simulink model "PMSM_FOC_CLOOP"  (R2022a)
settings: Solver=FixedStepAuto  StartTime=0.0  StopTime=0.5  FixedStep=Ts  RelTol=1e-3
undefined symbols (not defined in the file): Ki_C, Kp_C, pmsm, Ts
libraries: mcbcontrolslib x5, slpidlib x2, mcbplantlib x1, autolibpmsmexterior x1
settings Model: Creator=徐国强  LastModifiedBy=徐国强

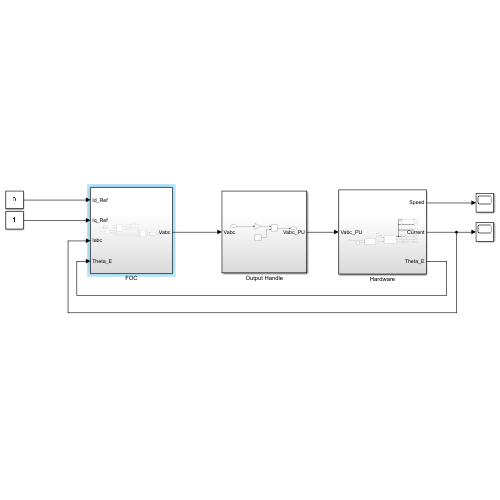
[thumbnail: Simulink's stored preview of the top-level diagram]
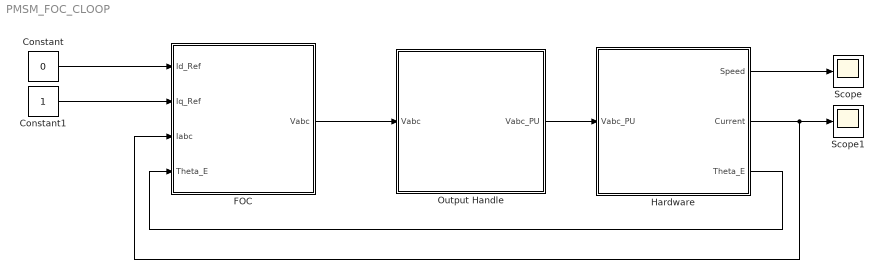
== system PMSM_FOC_CLOOP ==
  Constant : Constant  Value=0
  Constant1 : Constant
  FOC : Subsystem
  Hardware : Subsystem
  Output Handle : Subsystem
  Scope : Scope
  Scope1 : Scope
  wires:
  FOC/1(Vabc) -> Output Handle/1(Vabc)
  Output Handle/1(Vabc_PU) -> Hardware/1(Vabc_PU)
  Hardware/1(Speed) -> Scope/1
  Hardware/2(Current) -> FOC/3(Iabc), Scope1/1
  Hardware/3(Theta_E) -> FOC/4(Theta_E)
  Constant/1 -> FOC/1(Id_Ref)
  Constant1/1 -> FOC/2(Iq_Ref)

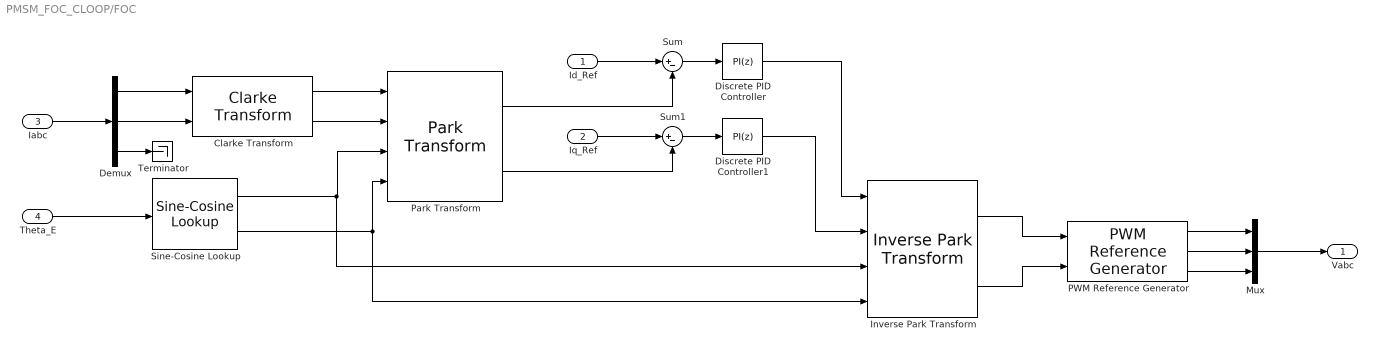
== system PMSM_FOC_CLOOP/FOC ==
  Id_Ref : Inport
  Iq_Ref : Inport  Port=2
  Iabc : Inport  Port=3
  Theta_E : Inport  Port=4
  Clarke Transform : mcbcontrolslib/Clarke Transform  VariantControl=Variant2
  Demux : Demux  Outputs=3
  Discrete PID Controller : slpidlib/PID Controller  Controller=PI  Form=Parallel  TimeDomain=Discrete-time  UseExternalTs=off  SampleTime=-1  IntegratorMethod=Forward Euler  FilterMethod=Forward Euler  ControllerParametersSource=internal  P=Kp_C  I=Ki_C  UseKiTs=off  D=0  N=100  UseFilter=on  TunerSelectOption=Transfer Function Based (PID Tuner App)  InitialConditionSource=internal  InitialConditionForIntegrator=0  InitialConditionForFilter=0  DifferentiatorICPrevScaledInput=0  ExternalReset=none  TrackingMode=off  Kt=1  LimitOutput=on  SatLimitsSource=internal  UpperSaturationLimit=12/sqrt(3)  LowerSaturationLimit=-12/sqrt(3)  LinearizeAsGain=off  AntiWindupMode=none  Kb=1  POutMin=[]  POutMax=[]  IOutMin=[]  IOutMax=[]  DOutMin=[]  DOutMax=[]  NOutMin=[]  NOutMax=[]  SumOutMin=[]  SumOutMax=[]  SaturationOutMin=[]  SaturationOutMax=[]  PParamMin=[]  PParamMax=[]  IParamMin=[]  IParamMax=[]  DParamMin=[]  DParamMax=[]  NParamMin=[]  NParamMax=[]  KbParamMin=[]  KbParamMax=[]  KtParamMin=[]  KtParamMax=[]  KbOutMin=[]  KbOutMax=[]  KtOutMin=[]  KtOutMax=[]  IntegratorOutMin=[]  IntegratorOutMax=[]  FilterOutMin=[]  FilterOutMax=[]  SumI1OutMin=[]  SumI1OutMax=[]  SumI2OutMin=[]  SumI2OutMax=[]  SumI3OutMin=[]  SumI3OutMax=[]  SumI4OutMin=[]  SumI4OutMax=[]  SumDOutMin=[]  SumDOutMax=[]  DifferentiatorOutMin=[]  DifferentiatorOutMax=[]  FilterDiffOutCoefMin=[]  FilterDiffOutCoefMax=[]  ReciprocalOutMin=[]  ReciprocalOutMax=[]  SumDenOutMin=[]  SumDenOutMax=[]  SumNumOutMin=[]  SumNumOutMax=[]  DivideOutMin=[]  DivideOutMax=[]  UdiffTsProdOutMin=[]  UdiffTsProdOutMax=[]  NTsProdOutMin=[]  NTsProdOutMax=[]  UintegralTsProdOutMin=[]  UintegralTsProdOutMax=[]  UngainTsProdOutMin=[]  UngainTsProdOutMax=[]  IntegratorContinuousStateAttributes=''  IntegratorStateMustResolveToSignalObject=off  IntegratorRTWStateStorageClass=Auto  FilterContinuousStateAttributes=''  FilterStateMustResolveToSignalObject=off  FilterRTWStateStorageClass=Auto  ParallelPVariant=InternalParameters  IdealPVariant=Disabled  IVariant=InternalParameters  DVariant=Disabled  IntegratorVariant=Discrete  SatVariant=Enabled  AWVariant=Passthrough  PCopyVariant=Disabled  TRVariant=Disabled  FdbkBlocksVariant=Forward  IdealPFdbkVariant=Disabled  SatFdbkVariant=Disabled  DerivativeFilterVariant=Disabled  NVariant=Disabled  NCopyVariant=Disabled_SignalSpec  FilterICVariant=Disabled  IntegratorICVariant=InternalICs  ExternalResetVariant=Disabled  TRSumVariant=Passthrough  SumFdbkVariant=Disabled  SumVariant=Sum_PI  TsampFilterVariant=InternalTs  TsampNgainVariant=Passthrough  TsampIntegralVariant=Passthrough  ExternalSaturationOutDataTypeStr=Inherit: Same as second input  aMode=0
  Discrete PID Controller1 : slpidlib/PID Controller  Controller=PI  Form=Parallel  TimeDomain=Discrete-time  UseExternalTs=off  SampleTime=-1  IntegratorMethod=Forward Euler  FilterMethod=Forward Euler  ControllerParametersSource=internal  P=Kp_C  I=Ki_C  UseKiTs=off  D=0  N=100  UseFilter=on  TunerSelectOption=Transfer Function Based (PID Tuner App)  InitialConditionSource=internal  InitialConditionForIntegrator=0  InitialConditionForFilter=0  DifferentiatorICPrevScaledInput=0  ExternalReset=none  TrackingMode=off  Kt=1  LimitOutput=on  SatLimitsSource=internal  UpperSaturationLimit=12/sqrt(3)  LowerSaturationLimit=-12/sqrt(3)  LinearizeAsGain=off  AntiWindupMode=none  Kb=1  POutMin=[]  POutMax=[]  IOutMin=[]  IOutMax=[]  DOutMin=[]  DOutMax=[]  NOutMin=[]  NOutMax=[]  SumOutMin=[]  SumOutMax=[]  SaturationOutMin=[]  SaturationOutMax=[]  PParamMin=[]  PParamMax=[]  IParamMin=[]  IParamMax=[]  DParamMin=[]  DParamMax=[]  NParamMin=[]  NParamMax=[]  KbParamMin=[]  KbParamMax=[]  KtParamMin=[]  KtParamMax=[]  KbOutMin=[]  KbOutMax=[]  KtOutMin=[]  KtOutMax=[]  IntegratorOutMin=[]  IntegratorOutMax=[]  FilterOutMin=[]  FilterOutMax=[]  SumI1OutMin=[]  SumI1OutMax=[]  SumI2OutMin=[]  SumI2OutMax=[]  SumI3OutMin=[]  SumI3OutMax=[]  SumI4OutMin=[]  SumI4OutMax=[]  SumDOutMin=[]  SumDOutMax=[]  DifferentiatorOutMin=[]  DifferentiatorOutMax=[]  FilterDiffOutCoefMin=[]  FilterDiffOutCoefMax=[]  ReciprocalOutMin=[]  ReciprocalOutMax=[]  SumDenOutMin=[]  SumDenOutMax=[]  SumNumOutMin=[]  SumNumOutMax=[]  DivideOutMin=[]  DivideOutMax=[]  UdiffTsProdOutMin=[]  UdiffTsProdOutMax=[]  NTsProdOutMin=[]  NTsProdOutMax=[]  UintegralTsProdOutMin=[]  UintegralTsProdOutMax=[]  UngainTsProdOutMin=[]  UngainTsProdOutMax=[]  IntegratorContinuousStateAttributes=''  IntegratorStateMustResolveToSignalObject=off  IntegratorRTWStateStorageClass=Auto  FilterContinuousStateAttributes=''  FilterStateMustResolveToSignalObject=off  FilterRTWStateStorageClass=Auto  ParallelPVariant=InternalParameters  IdealPVariant=Disabled  IVariant=InternalParameters  DVariant=Disabled  IntegratorVariant=Discrete  SatVariant=Enabled  AWVariant=Passthrough  PCopyVariant=Disabled  TRVariant=Disabled  FdbkBlocksVariant=Forward  IdealPFdbkVariant=Disabled  SatFdbkVariant=Disabled  DerivativeFilterVariant=Disabled  NVariant=Disabled  NCopyVariant=Disabled_SignalSpec  FilterICVariant=Disabled  IntegratorICVariant=InternalICs  ExternalResetVariant=Disabled  TRSumVariant=Passthrough  SumFdbkVariant=Disabled  SumVariant=Sum_PI  TsampFilterVariant=InternalTs  TsampNgainVariant=Passthrough  TsampIntegralVariant=Passthrough  ExternalSaturationOutDataTypeStr=Inherit: Same as second input  aMode=0
  Inverse Park Transform : mcbcontrolslib/Inverse Park Transform  AxisAlignment=D-axis
  Mux : Mux  Inputs=3
  PWM Reference Generator : mcbcontrolslib/PWM Reference Generator  inSignal=Valphabeta  modType=SVM: space vector modulation
      settings: SourceProductBaseCode=MT
  Park Transform : mcbcontrolslib/Park Transform  AxisAlignment=D-axis
      settings: SourceProductBaseCode=MT
  Sine-Cosine Lookup : mcbcontrolslib/Sine-Cosine Lookup  AngleInput=Radians  N_points=1024
      settings: SourceProductBaseCode=MT
  Sum : Sum  Inputs=|+-
  Sum1 : Sum  Inputs=|+-
  Terminator : Terminator
  Vabc : Outport
  wires:
  Theta_E/1 -> Sine-Cosine Lookup/1
  Mux/1 -> Vabc/1
  PWM Reference Generator/3 -> Mux/3
  PWM Reference Generator/2 -> Mux/2
  PWM Reference Generator/1 -> Mux/1
  Inverse Park Transform/2 -> PWM Reference Generator/2
  Inverse Park Transform/1 -> PWM Reference Generator/1
  Iabc/1 -> Demux/1
  Demux/3 -> Terminator/1
  Clarke Transform/1 -> Park Transform/1
  Sine-Cosine Lookup/1 -> Inverse Park Transform/3, Park Transform/3
  Sine-Cosine Lookup/2 -> Inverse Park Transform/4, Park Transform/4
  Id_Ref/1 -> Sum/1
  Park Transform/1 -> Sum/2
  Iq_Ref/1 -> Sum1/1
  Park Transform/2 -> Sum1/2
  Sum/1 -> Discrete PID Controller/1
  Sum1/1 -> Discrete PID Controller1/1
  Discrete PID Controller1/1 -> Inverse Park Transform/2
  Discrete PID Controller/1 -> Inverse Park Transform/1
  Clarke Transform/2 -> Park Transform/2
  Demux/1 -> Clarke Transform/1
  Demux/2 -> Clarke Transform/2

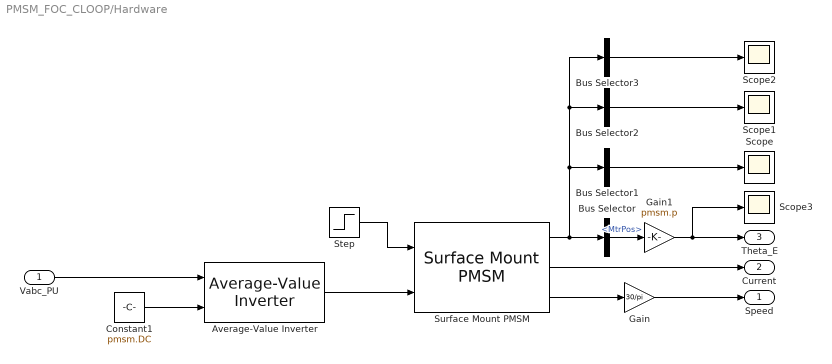
== system PMSM_FOC_CLOOP/Hardware ==
  Vabc_PU : Inport
  Average-Value Inverter : mcbplantlib/Average-Value Inverter
  Bus Selector : BusSelector  OutputSignals=MtrPos
  Bus Selector1 : BusSelector  OutputSignals=IdSync,IqSync  OutputAsBus=on
  Bus Selector2 : BusSelector  OutputSignals=VdSync,VqSync  OutputAsBus=on
  Bus Selector3 : BusSelector  OutputSignals=MtrTrq  OutputAsBus=on
  Constant1 : Constant  Value=pmsm.DC
  Gain : Gain  Gain=30/pi
  Gain1 : Gain  Gain=pmsm.p
  Scope{,1..3} (4 alike) : Scope
  Step : Step  Time=0.2  After=0.1*pmsm.T_rated  SampleTime=0
  Surface Mount PMSM : autolibpmsmexterior/Surface Mount PMSM  port_config=Torque  sim_type=Discrete  Ts=Ts  P=pmsm.p  Rs=pmsm.Rs  Ldq_=pmsm.Ld  KConstText=Permanent flux linkage constant (lambda_pm):  lambda_pm=pmsm.FluxPM  Ke=159.9771  Kt=1.323  mechanical=[pmsm.J, pmsm.B, 0]  idq0=[0 0]  theta_init=0  omega_init=0  KConst=pmsm.FluxPM  lambda_pm_calc=pmsm.FluxPM  RefBlkName='autolibpmsmexterior/Surface Mount PMSM'  aMode=5  Ldq="[0.0017      0.0017]"
      settings: SourceProductBaseCode=PW,DR,MT,VE
  Speed : Outport
  Current : Outport  Port=2
  Theta_E : Outport  Port=3
  wires:
  Vabc_PU/1 -> Average-Value Inverter/1
  Gain1/1 -> Scope3/1, Theta_E/1
  Step/1 -> Surface Mount PMSM/1
  Surface Mount PMSM/1 -> Bus Selector3/1, Bus Selector2/1, Bus Selector1/1, Bus Selector/1
  Surface Mount PMSM/3 -> Gain/1
  Average-Value Inverter/1 -> Surface Mount PMSM/2
  Surface Mount PMSM/2 -> Current/1
  Gain/1 -> Speed/1
  Constant1/1 -> Average-Value Inverter/2
  Bus Selector/1 -> Gain1/1  "<MtrPos>"
  Bus Selector1/1 -> Scope/1
  Bus Selector2/1 -> Scope1/1
  Bus Selector3/1 -> Scope2/1

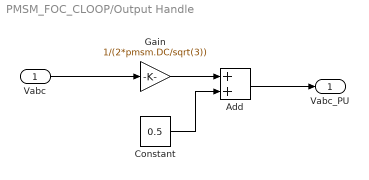
== system PMSM_FOC_CLOOP/Output Handle ==
  Vabc : Inport
  Add : Sum
  Constant : Constant  Value=0.5
  Gain : Gain  Gain=1/(2*pmsm.DC/sqrt(3))
  Vabc_PU : Outport
  wires:
  Constant/1 -> Add/2
  Add/1 -> Vabc_PU/1
  Gain/1 -> Add/1
  Vabc/1 -> Gain/1
